simulink subsystem "encoder_distancia"  (R2023b)
settings: Solver=VariableStepAuto  StartTime=0.0  StopTime=10.0  RelTol=1e-3
libraries: arduinosensorlib x2
settings Model: Creator=Usuario_UMA  LastModifiedBy=Manuel

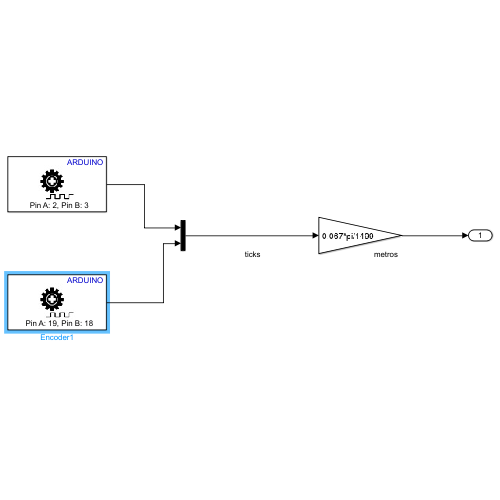
[thumbnail: Simulink's stored preview of the top-level diagram]
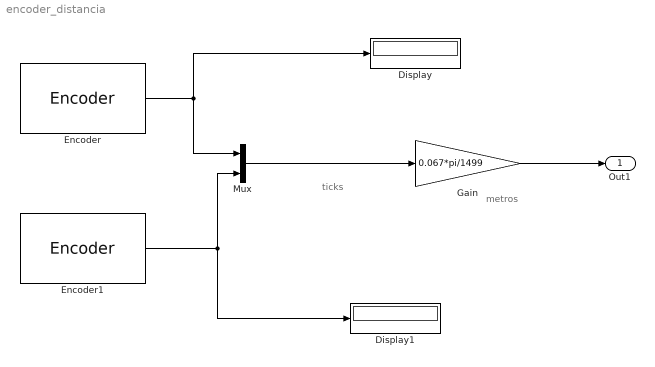
== system encoder_distancia ==
  note: metros
  note: ticks
  Display : Display
  Display1 : Display
  Encoder : arduinosensorlib/Encoder  InputA=2  InputB=3  Mode=No reset  SampleTime=-1
  Encoder1 : arduinosensorlib/Encoder  InputA=19  InputB=18  Mode=No reset  SampleTime=-1
  Gain : Gain  Gain=0.067*pi/1499  ParamDataTypeStr=double
  Mux : Mux  Inputs=2
  Out1 : Outport
  wires:
  Encoder/1 -> Display/1, Mux/1
  Encoder1/1 -> Display1/1, Mux/2
  Mux/1 -> Gain/1
  Gain/1 -> Out1/1
